simulink model "otk_ut"  (Simulink 8.1)
settings: Solver=FixedStepDiscrete  StartTime=0.0  StopTime=10.0  FixedStep=0.005  RelTol=1e-3
libraries: siltestlib x7, otk x1
settings Model: Creator=AT015555  LastModifiedBy=AT015555
settings DataIOCC: SignalLoggingSaveFormat=Dataset
settings OptimizationCC: ExpressionDepthLimit=128
settings DebuggingCC: FcnCallInpInsideContextMsg=EnableAllAsError
settings GRTTargetCC: CombineOutputUpdateFcns=on  GRTInterface=off

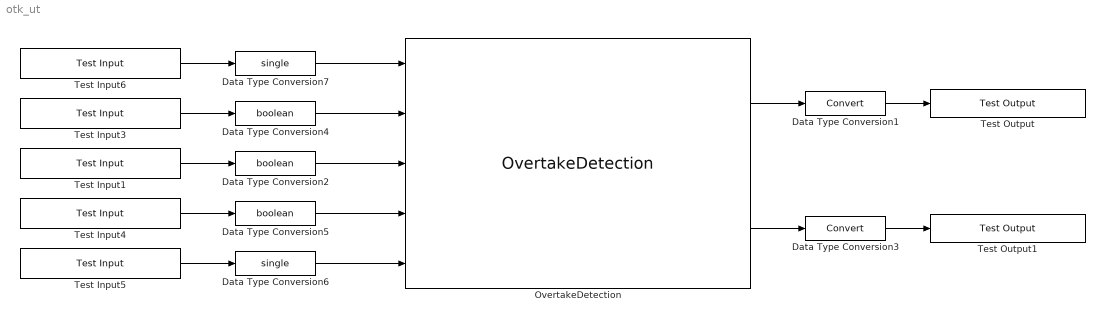
== system otk_ut ==
  Data Type Conversion1 : DataTypeConversion
  Data Type Conversion2 : DataTypeConversion  OutDataTypeStr=boolean
  Data Type Conversion3 : DataTypeConversion
  Data Type Conversion4 : DataTypeConversion  OutDataTypeStr=boolean
  Data Type Conversion5 : DataTypeConversion  OutDataTypeStr=boolean
  Data Type Conversion6 : DataTypeConversion  OutDataTypeStr=single
  Data Type Conversion7 : DataTypeConversion  OutDataTypeStr=single
  OvertakeDetection : otk/OvertakeDetection
  Test Input1 : siltestlib/Test Input  varname=VDINR_TurnSignalSwR_flg  sampletime=0.005
  Test Input3 : siltestlib/Test Input  varname=VDINR_TurnSignalSwL_flg  sampletime=0.005
  Test Input4 : siltestlib/Test Input  varname=VIFO_ACCTargetVehAssigned_flg  sampletime=0.005
  Test Input5 : siltestlib/Test Input  varname=VJUD_ACCSetSpeedPrev_kph  sampletime=0.005
  Test Input6 : siltestlib/Test Input  varname=VIFO_VehSpd_kph  sampletime=0.005
  Test Output : siltestlib/Test Output  varname=VIFO_DriverOvertakeReq_flg  sampletime=-1
  Test Output1 : siltestlib/Test Output  varname=VIFO_DriverTurnSignalOn_flg  sampletime=-1
  wires:
  Test Input6/1 -> Data Type Conversion7/1
  OvertakeDetection/1 -> Data Type Conversion1/1
  Data Type Conversion1/1 -> Test Output/1
  Data Type Conversion7/1 -> OvertakeDetection/1
  Test Input3/1 -> Data Type Conversion4/1
  Data Type Conversion4/1 -> OvertakeDetection/2
  Test Input4/1 -> Data Type Conversion5/1
  Data Type Conversion5/1 -> OvertakeDetection/4
  Test Input5/1 -> Data Type Conversion6/1
  Data Type Conversion6/1 -> OvertakeDetection/5
  Test Input1/1 -> Data Type Conversion2/1
  Data Type Conversion2/1 -> OvertakeDetection/3
  Data Type Conversion3/1 -> Test Output1/1
  OvertakeDetection/2 -> Data Type Conversion3/1
